simulink model "sl_solarcell"  (R2014a)
settings: Solver=ode23tb  StartTime=0.0  StopTime=10  RelTol=1e-4
undefined symbols (not defined in the file or in its folder): Ts
libraries: powerlib x8, simulink x3, simulink_extras x2
settings Model: Creator=cosorio  LastModifiedBy=cosorio
settings DataIOCC: LimitDataPoints=off  SignalLoggingSaveFormat=ModelDataLogs  SaveOutput=off  SignalLogging=off  SaveTime=off
settings OptimizationCC: ExpressionDepthLimit=2147483647
settings DebuggingCC: UnderspecifiedInitializationDetection=Classic  SolverPrmCheckMsg=none  FcnCallInpInsideContextMsg=UseLocalSettings  StateNameClashWarn=warning
settings GRTTargetCC: CombineOutputUpdateFcns=off  GRTInterface=on

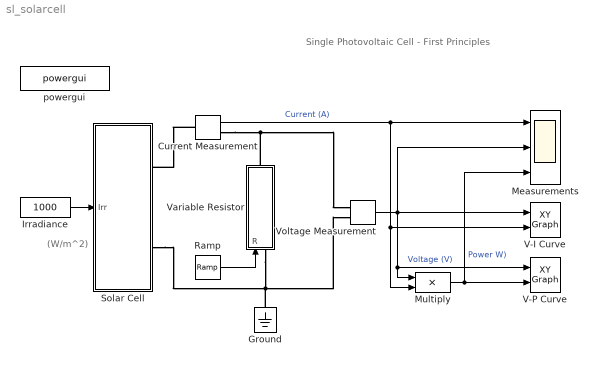
== system sl_solarcell ==
  note: Single Photovoltaic Cell - First Principles
  note: (W/m^2)
  Current Measurement : powerlib/Measurements/Current Measurement  PhasorSimulation=off  OutputType=Complex  PSBequivalent=0
  Ground : powerlib/Elements/Ground  LConnTagsString=a
  Irradiance : Constant  Value=1000
  Measurements : Scope  NumInputPorts=3
      settings: YMin=0~0~0  YMax=6~1~3  SaveName=SLSolarCellData
  Multiply : Product  Inputs=**
  Ramp : simulink/Sources/Ramp  slope=0.1  start=0  X0=0
  Solar Cell : Subsystem  mask(Solar Cell){Isc=5, Voc=0.6, Ir0=1000, N=1.5, Rs=0.001, Rp=1000, tau=1e-04, Io=5}
      mask prompts: Isc "Short-circuit current, Isc (A):"; Voc "Open-circuit voltage, Voc (V):"; Ir0 "Irradiance used for measurements, Ir0 (W/m2):"; N "Quality factor, N:"; Rs "Series resistance, Rs (ohms):"; Rp "Parallel resistance, Rp (ohms):"; tau "Time constant (sec):"; Io "Initial current output (A):"
      mask help:
      | Simulink implementation of an idividual solar cell. The cell is modelled as a parallel combination of a current source, an exponential diode and an internal resistance Rp, connected in series with a resistance Rs.
      | The cell output current is given by:
      |
      | Ipv = Iph - Is * (exp((V + I*Rs)/(N*Vt)) - 1) - (V + I*Rs)/Rp
      |
      | Where Iph is the solar irradiance generated current, Is is the diode saturation current, Vt is the thermal voltage, N is the diode quality factor (emission coefficient).
      | The calculations are performed at a fixed operating temperature of 25 oC.
      |
      | A first order transfer function is used to break the algebraic loop. The time constant of this transfer function should be adjusted such that it will not significantly affect your model dynamics.
      mask init:
      | %% Cell thermal voltage calculation
      | T = 25 + 273;   % Device operating temperature (oC)
      | k = 1.3806e-23; % Boltzman constant (J/oK)
      | q = 1.602e-19;  % Elementary charge on an electron (oC)
      | Vt = k*T/q;     % Thermal voltage
      | 
      | %% Diode saturation current calculation
      | Is = Isc/(exp(Voc/(N*Vt))-1);
  V-I Curve : simulink/Sinks/XY Graph  xmin=0  xmax=0.6  ymin=0  ymax=6  st=-1
  V-P Curve : simulink/Sinks/XY Graph  xmin=0  xmax=0.6  ymin=0  ymax=3  st=-1
  Variable Resistor : Subsystem  mask(Variable Resistor){tau=1e-4, I0out=5, I0in=0}
      mask prompts: tau "Time constant (sec):"; I0out "Initial Output Current (A):"; I0in "Initial Input Current (A):"
      mask help: This block implements a SimPowerSystems variable resistor using Simulink
  Voltage Measurement : powerlib/Measurements/Voltage Measurement  PhasorSimulation=off  OutputType=Complex  PSBequivalent=0
  powergui : powerlib/powergui  Priority=1  SimulationMode=Continuous  SolverType=Tustin  SampleTime=Ts  frequency=60  SPID=off  DisableSnubberDevices=off  DisableRonSwitches=off  DisableVfSwitches=off  SwTol=0  Interpol=off  DisplayEquations=off  Ts=0  methode=off  frequencyindice=0  Pbase=100e6  ErrMax=1e-4  Iterations=50  UnitsV=kV  UnitsW=MW  FunctionMessages=off  echomessages=off  HookPort=off  EnableUseOfTLC=off  x0status=blocks  RestoreLinks=warning  ResistiveCurrentMeasurement=off  Frange=[0:2:500]  Ylog=off  Xlog=on  ShowGrid=off  save=off  variable=ZData  structure=0  ZoomFFT=on  StartTime=0.0  cycles=1  DisplayStyle=1  fundamental=60  FreqAxis=off  MaxFrequency=1000  frequencyindicesteady=1  RmsSteady=1  display=off
  wires:
  Irradiance/1 -> Solar Cell/1(Irr)
  Current Measurement/1 -> Measurements/1, V-I Curve/2, Multiply/2  "Current (A)"
  Voltage Measurement/1 -> V-I Curve/1, Multiply/1, V-P Curve/1, Measurements/2  "Voltage (V)"
  Multiply/1 -> V-P Curve/2, Measurements/3  "Power W)"
  Ramp/1 -> Variable Resistor/1(R)
  connections:
  Solar Cell/RConn2 -- Variable Resistor/LConn1 -- Voltage Measurement/LConn2 -- Ground/LConn1
  Current Measurement/RConn1 -- Variable Resistor/RConn1 -- Voltage Measurement/LConn1
  Current Measurement/LConn1 -- Solar Cell/RConn1

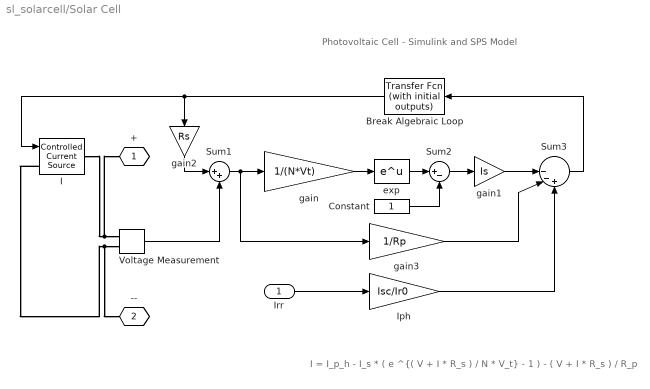
== system sl_solarcell/Solar Cell ==
  note: I = I_p_h - I_s * ( e ^{( V + I * R_s ) / N * V_t} - 1 ) - ( V + I * R_s ) / R_p
  note: Photovoltaic Cell - Simulink and SPS Model
  Irr : Inport
  Break Algebraic Loop : simulink_extras/Additional Linear/Transfer Fcn (with initial outputs)  N=[1]  D="[tau  1]"  Y0=Io  U0=0
  Constant : Constant
  I : powerlib/Electrical Sources/Controlled Current Source  Initialize=on  Source_Type=DC  Amplitude=5  Phase=0  Frequency=0  Measurements=None
  Iph : Gain  Gain=Isc/Ir0
  Sum1 : Sum  Inputs=|++
  Sum2 : Sum  Inputs=|+-
  Sum3 : Sum  Inputs=||--+
  Voltage Measurement : powerlib/Measurements/Voltage Measurement  PhasorSimulation=off  OutputType=Complex  PSBequivalent=0
  exp : Math  SaturateOnIntegerOverflow=on
  gain : Gain  Gain=1/(N*Vt)
  gain1 : Gain  Gain=Is
  gain2 : Gain  Gain=Rs
  gain3 : Gain  Gain=1/Rp
  + : PMIOPort  Tag=PMCPort  Port=1  Side=Right
  -- : PMIOPort  Tag=PMCPort  Port=2  Side=Right
  wires:
  Sum2/1 -> gain1/1
  Constant/1 -> Sum2/2
  exp/1 -> Sum2/1
  Sum1/1 -> gain/1, gain3/1
  gain/1 -> exp/1
  Sum3/1 -> Break Algebraic Loop/1
  Voltage Measurement/1 -> Sum1/2
  Irr/1 -> Iph/1
  Break Algebraic Loop/1 -> gain2/1, I/1
  gain2/1 -> Sum1/1
  gain1/1 -> Sum3/1
  gain3/1 -> Sum3/2
  Iph/1 -> Sum3/3
  connections:
  Voltage Measurement/LConn1 -- +/RConn1 -- I/RConn1
  Voltage Measurement/LConn2 -- --/RConn1 -- I/LConn1

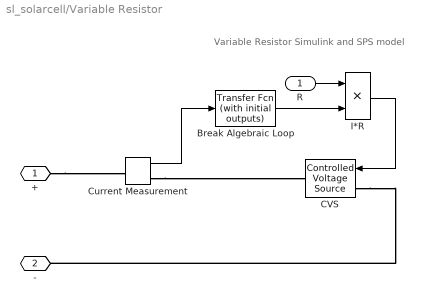
== system sl_solarcell/Variable Resistor ==
  note: Variable Resistor Simulink and SPS model
  R : Inport
  Break Algebraic Loop : simulink_extras/Additional Linear/Transfer Fcn (with initial outputs)  N=[1]  D="[tau  1]"  Y0=I0out  U0=I0in
  CVS : powerlib/Electrical Sources/Controlled Voltage Source  Initialize=on  Source_Type=AC  Amplitude=0  Phase=0  Frequency=0  Measurements=None
  Current Measurement : powerlib/Measurements/Current Measurement  PhasorSimulation=off  OutputType=Complex  PSBequivalent=0
  I*R : Product  Inputs=**
  + : PMIOPort  Port=1  Side=Right
  - : PMIOPort  Port=2  Side=Left
  wires:
  I*R/1 -> CVS/1
  Current Measurement/1 -> Break Algebraic Loop/1
  Break Algebraic Loop/1 -> I*R/2
  R/1 -> I*R/1
  connections:
  Current Measurement/RConn1 -- CVS/RConn1
  +/RConn1 -- Current Measurement/LConn1
  CVS/LConn1 -- -/RConn1
